simulink model "test_controller_with_filter"  (R2020a)
settings: Solver=VariableStepAuto  StartTime=0.0  StopTime=2  MaxStep=1e-3  RelTol=1e-3
settings Model: Creator=james  LastModifiedBy=james

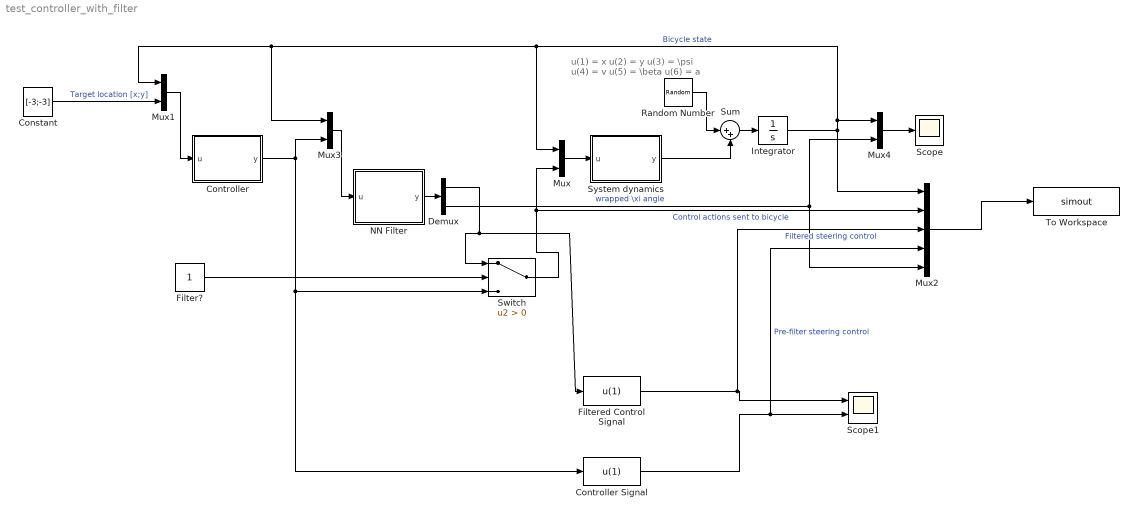
== system test_controller_with_filter ==
  note: u(1) = x
      | u(2) = y
      | u(3) = \psi
      | u(4) = v
      | u(5) = \beta
      | u(6) = a
  Constant : Constant  Value=[-3;-3]
  Controller : MATLAB Function  TreatAsAtomicUnit=on
  Controller Signal : Fcn  Expr=u(1)
  Demux : Demux  Outputs=[2;1]
  Filter? : Constant
  Filtered Control Signal : Fcn  Expr=u(1)
  Integrator : Integrator  InitialCondition=[2;2;2.5*pi/3;3]
  Mux : Mux  Inputs=[4;2]
  Mux1 : Mux  Inputs=[4;2]
  Mux2 : Mux  Inputs=[4;2;1;1;1]
  Mux3 : Mux  Inputs=[4;2]
  Mux4 : Mux  Inputs=2
  NN Filter : MATLAB Function  TreatAsAtomicUnit=on
  Random Number : RandomNumber  Mean=[0;0;0;0]  Variance=[0;0;0;0]  SampleTime=0.001
  Scope : Scope
  Scope1 : Scope  NumInputPorts=2
  Sum : Sum  Inputs=|++
  Switch : Switch  Criteria=u2 > Threshold
  System dynamics : MATLAB Function  TreatAsAtomicUnit=on
  To Workspace : ToWorkspace  VariableName=simout  SaveFormat=Timeseries  SampleTime=-1
  wires:
  Integrator/1 -> Mux4/1, Mux/1, Mux3/1, Mux1/1, Mux2/1  "Bicycle state"
  Constant/1 -> Mux1/2  "Target location [x;y]"
  Mux/1 -> System dynamics/1(u)
  Switch/1 -> Mux/2, Mux2/2  "Control actions sent to bicycle"
  Mux1/1 -> Controller/1(u)
  Mux2/1 -> To Workspace/1
  System dynamics/1(y) -> Sum/2
  Sum/1 -> Integrator/1
  Random Number/1 -> Sum/1
  Filter?/1 -> Switch/2
  Controller/1(y) -> Controller Signal/1, Switch/3, Mux3/2
  Mux3/1 -> NN Filter/1(u)
  Demux/1 -> Switch/1, Filtered Control Signal/1
  Filtered Control Signal/1 -> Mux2/3, Scope1/1  "Filtered steering control"
  Controller Signal/1 -> Mux2/4, Scope1/2  "Pre-filter steering control"
  NN Filter/1(y) -> Demux/1
  Mux4/1 -> Scope/1
  Demux/2 -> Mux2/5, Mux4/2  "wrapped \\xi angle"

== matlab function test_controller_with_filter/Controller ==
  data: u input; y output
function y = fcn(u)

% u(1) = x
% u(2) = y
% u(3) = \psi
% u(4) = v
% u(5) = target location x
% u(6) = target location y

% targetAngle = atan2((-u(6)+u(2)),(-u(5)+u(1)));
% 
% if targetAngle >= 0 && targetAngle <= pi/2
%     targetAngle = -pi+targetAngle;    
% elseif targetAngle > pi/2 && targetAngle <= pi
%     targetAngle = -targetAngle;
% elseif targetAngle < 0 && targetAngle >= -pi/2
%     targetAngle = pi-targetAngle;
% else
%     targetAngle = pi + targetAngle;
% end

targetAngle = atan2((u(6)-u(2)),(u(5)-u(1)));


% ==== Get the state angle in the range [-pi,pi] ====

% First get the state angle into the range [-2*pi,2*pi]
wrappedStateAngle = u(3) - fix(u(3)/(2*pi))*(2*pi);
% Correct angles with abs larger than pi:
if wrappedStateAngle >= pi
    wrappedStateAngle = wrappedStateAngle - 2*pi;
end
if wrappedStateAngle <= -pi
    wrappedStateAngle = 2*pi + wrappedStateAngle;
end

% gainSign = 1;
% if targetAngle >=0 && wrappedStateAngle <= 0
%     gainSign = -1;
% end
% if targetAngle <=0 && wrappedStateAngle >= 0
%     gainSign = 1;
% end
% gainSign = -1;

gainSign = 1;
if (targetAngle >=0 && wrappedStateAngle <= 0 && wrappedStateAngle <= -targetAngle) || ...
        (targetAngle <=0 && wrappedStateAngle >= 0 && wrappedStateAngle >= -targetAngle)
    gainSign = -1;
end

controlinput = gainSign*2*(targetAngle-wrappedStateAngle);
if controlinput > pi/4
    controlinput = pi/4;
elseif controlinput < -pi/4
    controlinput = -pi/4;
end
y = [atan(0.5*tan(controlinput));0];

== matlab function test_controller_with_filter/System dynamics ==
  data: u input; y output
function y = fcn(u)

y = [u(4)*cos(u(3)+u(5)); u(4)*sin(u(3)+u(5)); (1/0.23)*u(4)*sin(u(5));u(6)];

== matlab function test_controller_with_filter/NN Filter ==
  data: u input; y output
function y = fcn(u)

% ============================ !! IMPORTANT !! ============================
% 'THRESH.M' ***MUST*** BE IN THE MATLAB PATH OR THE CURRENT FOLDER BEFORE
% RUNNING THIS MODEL!!
% =========================================================================


% 'coder.extern' tells simulink that 'thresh1' and 'thresh2' are external 
% functions, and should be handled by the MATLAB interpreter
coder.extrinsic('thresh');

% These zero assignments are NECESSARY, so that MATLAB knows the type of 
% these variables:
y=[0;0;0];
lower = 0;
upper = 0;
control = 0;

rBar = 2; % Mimum physical distance to origin
sigma = 0.25; % Parameter of the barrier function
barrier = @(xi) ( ...
		rBar./(sigma.*cos(xi/2) + 1 - sigma) ...
	);

wrappedPsi = u(3) - fix(u(3)/(2*pi))*(2*pi);
% Correct angles with abs() larger than pi:
if wrappedPsi <= 0
    wrappedPsi = 2*pi + wrappedPsi;
end

wrappedGamma = atan2(u(2),u(1)) - fix(atan2(u(2),u(1))/(2*pi))*(2*pi);
% Correct angles with abs() larger than pi:
if wrappedGamma <= 0
    wrappedGamma = 2*pi + wrappedGamma;
end


xi = wrappedGamma-wrappedPsi;
wrappedXi = xi - fix(xi/(2*pi))*(2*pi);
% Correct angles with abs() larger than pi:
if wrappedXi >= pi
    wrappedXi = wrappedXi - 2*pi;
end
if wrappedXi <= -pi
    wrappedXi = 2*pi + wrappedXi;
end

if sqrt(u(1)^2 + u(2)^2) > barrier(wrappedXi) + 0.7 % free control threshold
    y = [u(5);u(6);wrappedXi]; % Pass the steering control, u(5), unaltered
else
    idx = 1; % index variable to select NN
    control = u(5); % variable to store the control action we eventually use
    
    % Determin which NN we should use, based on the distance from the
    % origin and the orientation of the bicycle, xi:
    if sqrt(u(1)^2 + u(2)^2) >= barrier(wrappedXi) + 0.5
        idx = 3;
    elseif sqrt(u(1)^2 + u(2)^2) >= barrier(wrappedXi) + 0.25
        idx = 2;
    elseif sqrt(u(1)^2 + u(2)^2) >= barrier(wrappedXi)
        idx = 1;
    end

    %control = double(thresh(u(1),u(2),u(3),u(5),idx));
    control = double(thresh(u(1),u(2),wrappedXi,u(5),idx));
    
    y = [control;u(6);wrappedXi];
end
